simulink model "la01"  (R2017a)
settings: Solver=VariableStepAuto  StartTime=0.0  StopTime=0.1  RelTol=1e-3
libraries: dspsnks4 x1, dspsrcs4 x1
settings Model: Creator=HP  LastModifiedBy=HP

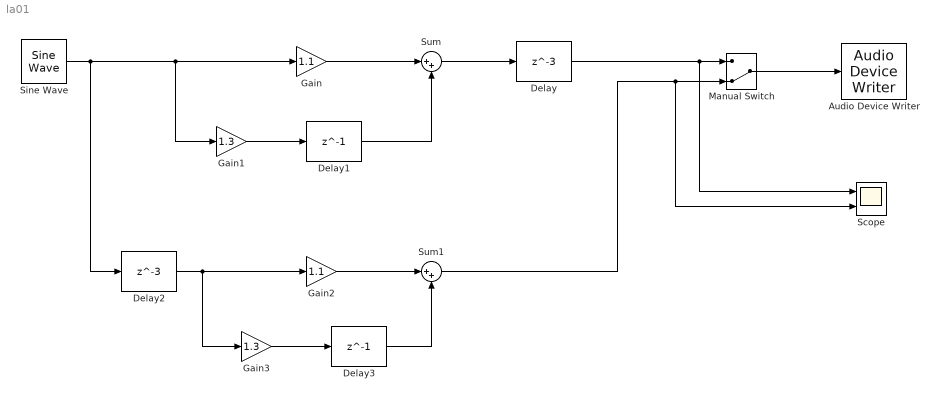
== system la01 ==
  Audio Device Writer : dspsnks4/Audio Device Writer  Driver=DirectSound  Device=Default  InheritSampleRate=on  SampleRate=44100  BitDepth=16-bit integer  BufferSize=4096  NumBuffers=10  DefaultOutputChannelMapping=on  OutputChannelMapping=1:2  OutputNumUnderrunSamples=off  DriverIdx=1  DeviceWarnFlag=''
  Delay : Delay  DelayLength=3  InputProcessing=Columns as channels (frame based)
  Delay1 : Delay  DelayLength=1  InputProcessing=Columns as channels (frame based)
  Delay2 : Delay  DelayLength=3  InputProcessing=Columns as channels (frame based)
  Delay3 : Delay  DelayLength=1  InputProcessing=Columns as channels (frame based)
  Gain : Gain  Gain=1.1
  Gain1 : Gain  Gain=1.3
  Gain2 : Gain  Gain=1.1
  Gain3 : Gain  Gain=1.3
  Manual Switch : ManualSwitch  CurrentSetting=0
  Scope : Scope  NumInputPorts=2
  Sine Wave : dspsrcs4/Sine Wave  Amplitude=1  Frequency=100  Phase=0  SampleMode=Discrete  OutComplex=Real  CompMethod=Trigonometric fcn  TableSize=Speed  SampleTime=1/1000  SamplesPerFrame=1  ResetState=Restart at time zero  OutputFrames=off  dataType=double  wordLen=16  udDataType=sfix(16)  fracBitsMode=Best precision  numFracBits=15  OutDataTypeStr=double  LastOutDataTypeStr=double
  Sum : Sum  Inputs=|++
  Sum1 : Sum  Inputs=|++
  wires:
  Manual Switch/1 -> Audio Device Writer/1
  Delay/1 -> Scope/1, Manual Switch/1
  Sum/1 -> Delay/1
  Gain/1 -> Sum/1
  Sine Wave/1 -> Delay2/1, Gain1/1, Gain/1
  Gain1/1 -> Delay1/1
  Delay1/1 -> Sum/2
  Gain2/1 -> Sum1/1
  Sum1/1 -> Scope/2, Manual Switch/2
  Gain3/1 -> Delay3/1
  Delay3/1 -> Sum1/2
  Delay2/1 -> Gain3/1, Gain2/1
